simulink model "zad3_3_1_c"  (Simulink 6.5)
settings: Solver=ode45  StartTime=0.0  StopTime=10.0  RelTol=1e-3
settings Model: Creator=rr44283  LastModifiedBy=rr44283

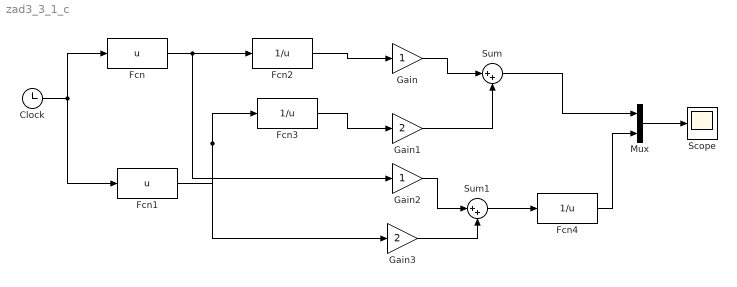
== system zad3_3_1_c ==
  Clock : Clock
      settings: Decimation=10
  Fcn : Fcn  Expr=u
  Fcn1 : Fcn  Expr=u
  Fcn2 : Fcn  Expr=1/u
  Fcn3 : Fcn  Expr=1/u
  Fcn4 : Fcn  Expr=1/u
  Gain : Gain
  Gain1 : Gain  Gain=2
  Gain2 : Gain
  Gain3 : Gain  Gain=2
  Mux : Mux  Inputs=2
  Scope : Scope
  Sum : Sum  Inputs=|++
  Sum1 : Sum  Inputs=|++
  wires:
  Fcn/1 -> Fcn2/1, Gain2/1
  Fcn1/1 -> Fcn3/1, Gain3/1
  Fcn3/1 -> Gain1/1
  Fcn2/1 -> Gain/1
  Gain1/1 -> Sum/2
  Gain/1 -> Sum/1
  Gain2/1 -> Sum1/1
  Gain3/1 -> Sum1/2
  Sum1/1 -> Fcn4/1
  Clock/1 -> Fcn/1, Fcn1/1
  Sum/1 -> Mux/1
  Fcn4/1 -> Mux/2
  Mux/1 -> Scope/1
